simulink model "PMSM_simulink"  (R2023b)
settings: Solver=VariableStepAuto  StartTime=0.0  StopTime=15  RelTol=1e-3
undefined symbols (not defined in the file or in its folder): dyn, foc, fw, load, lut, org, pmsm, sigbuilder_block
libraries: slpidlib x3, eeTransforms x2
settings Model: Creator=MatlabStation  LastModifiedBy=arne.spiessens
settings OptimizationCC: ReuseModelBlockBuffer=off
settings DebuggingCC: AlgebraicLoopMsg=none  ParameterPrecisionLossMsg=none

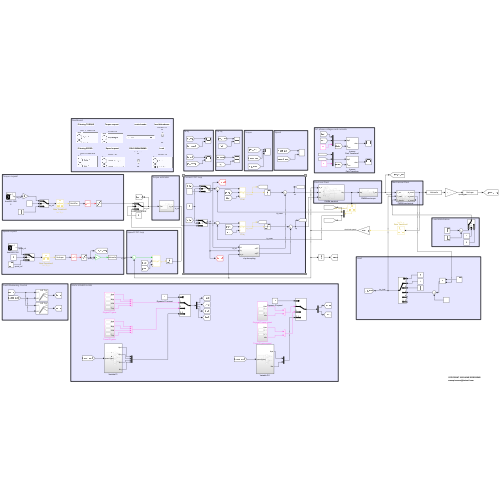
[thumbnail: Simulink's stored preview of the top-level diagram]
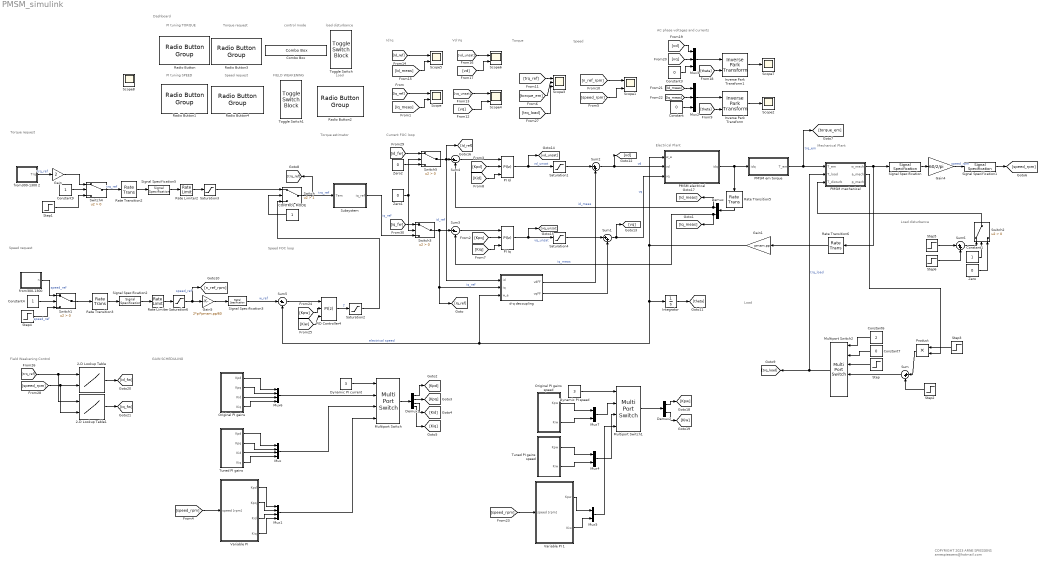
== system PMSM_simulink ==
  note: COPYRIGHT 2023 ARNE SPIESSENS
      | arnespiessens@hotmail.com
  note: Field Weakening Control
  note: Torque estimator
  note: Dashboard
  note: Load disturbance
  note: Speed FOC loop
  note: Speed request
  note: Torque request
  note: Current FOC loop
  note: Load
  note: GAIN SCHEDULING
  note: AC phase voltages and currents
  note: Speed
  note: Torque
  note: Vd Vq
  note: Id Iq
  note: Mechanical Plant
  note: Electrical Plant
  note: PI tuning TORQUE
  note: control mode
  note: PI tuning SPEED
  note: Torque request
  note: Speed request
  note: Load
  note: load disturbance
  note: FIELD WEAKENING
  2-D Lookup Table : Lookup_n-D  BreakpointsForDimension1=lut.trqLUT  BreakpointsForDimension2=lut.speedLUT  Table=lut.idLUT  InternalRulePriority=Speed  RndMeth=Simplest
      settings: InputPortMap=u0,u1
  2-D Lookup Table1 : Lookup_n-D  BreakpointsForDimension1=lut.trqLUT  BreakpointsForDimension2=lut.speedLUT  Table=lut.iqLUT  InternalRulePriority=Speed  RndMeth=Simplest
      settings: InputPortMap=u0,u1
  CONTROL MODE : Constant
  Combo Box : ComboBox  LabelPosition=Hide  SelectedLabel=Speed CL
      settings: Values={{'Torque CL', 'Speed CL'}, [2 1]}
  Constant : Constant  Value=0
  Constant1 : Constant
  Constant3 : Constant  Value=0
  Constant4 : Constant
  Constant6 : Constant  Value=2
  Constant7 : Constant  Value=0
  Constant9 : Constant
  Demux : Demux  Outputs=2
  Demux1 : Demux
  Demux2 : Demux  Outputs=2
  Dynamic PI current : Constant  Value=3
  Dynamic PI speed : Constant  Value=3
  Gain : Gain  Gain=2
  Gain1 : Gain  Gain=pmsm.pp
  Gain4 : Gain  Gain=60/2/pi
  Gain5 : Gain  Gain=2*pi*pmsm.pp/60
  Integrator : Integrator
  Inverse Park Transform : eeTransforms/Inverse Park Transform  AxisAlignment=Q-axis  PowerInvariant=off
      settings: LibrarySourceBlock=|
      | ee_sl_lib/Mathematical
      | Transforms/Inverse
      | Park Transform
  Inverse Park Transform1 : eeTransforms/Inverse Park Transform  AxisAlignment=Q-axis  PowerInvariant=off
      settings: LibrarySourceBlock=|
      | ee_sl_lib/Mathematical
      | Transforms/Inverse
      | Park Transform
  Multiport Switch : MultiPortSwitch  SaturateOnIntegerOverflow=off  InputSameDT=off
  Multiport Switch1 : MultiPortSwitch  SaturateOnIntegerOverflow=off  InputSameDT=off
  Multiport Switch2 : MultiPortSwitch  Inputs=5  SaturateOnIntegerOverflow=off  InputSameDT=off
  Mux : Mux
  Mux1 : Mux
  Mux2 : Mux  Inputs=3
  Mux3 : Mux  Inputs=3
  Mux4 : Mux  Inputs=2
  Mux5 : Mux  Inputs=2
  Mux6 : Mux
  Mux7 : Mux  Inputs=2
  Original PI gains : Subsystem
  Original PI gains speed : Subsystem
  PI Id : slpidlib/PID Controller  Controller=PI  Form=Parallel  TimeDomain=Discrete-time  UseExternalTs=off  SampleTime=foc.Ts_c  IntegratorMethod=Forward Euler  FilterMethod=Forward Euler  ControllerParametersSource=external  P=foc.Kpd  I=foc.Kid  UseKiTs=off  D=0  N=100  UseFilter=on  TunerSelectOption=Transfer Function Based (PID Tuner App)  InitialConditionSource=internal  InitialConditionForIntegrator=0  InitialConditionForFilter=0  DifferentiatorICPrevScaledInput=0  ExternalReset=none  TrackingMode=off  Kt=1  LimitOutput=on  SatLimitsSource=internal  UpperSaturationLimit=inf  LowerSaturationLimit=-inf  LinearizeAsGain=on  AntiWindupMode=clamping  Kb=foc.Kbd  LimitIntegrator=off  UpperIntegratorSaturationLimit=inf  LowerIntegratorSaturationLimit=-inf  POutMin=[]  POutMax=[]  IOutMin=[]  IOutMax=[]  DOutMin=[]  DOutMax=[]  NOutMin=[]  NOutMax=[]  SumOutMin=[]  SumOutMax=[]  SaturationOutMin=[]  SaturationOutMax=[]  PParamMin=[]  PParamMax=[]  IParamMin=[]  IParamMax=[]  DParamMin=[]  DParamMax=[]  NParamMin=[]  NParamMax=[]  KbParamMin=[]  KbParamMax=[]  KtParamMin=[]  KtParamMax=[]  KbOutMin=[]  KbOutMax=[]  KtOutMin=[]  KtOutMax=[]  IntegratorOutMin=[]  IntegratorOutMax=[]  FilterOutMin=[]  FilterOutMax=[]  SumI1OutMin=[]  SumI1OutMax=[]  SumI2OutMin=[]  SumI2OutMax=[]  SumI3OutMin=[]  SumI3OutMax=[]  SumI4OutMin=[]  SumI4OutMax=[]  SumDOutMin=[]  SumDOutMax=[]  DifferentiatorOutMin=[]  DifferentiatorOutMax=[]  FilterDiffOutCoefMin=[]  FilterDiffOutCoefMax=[]  ReciprocalOutMin=[]  ReciprocalOutMax=[]  SumDenOutMin=[]  SumDenOutMax=[]  SumNumOutMin=[]  SumNumOutMax=[]  DivideOutMin=[]  DivideOutMax=[]  UdiffTsProdOutMin=[]  UdiffTsProdOutMax=[]  NTsProdOutMin=[]  NTsProdOutMax=[]  UintegralTsProdOutMin=[]  UintegralTsProdOutMax=[]  UngainTsProdOutMin=[]  UngainTsProdOutMax=[]  ClampingZeroOutDataTypeStr=Inherit: Inherit via back propagation  ClampingZeroOutMin=[]  ClampingZeroOutMax=[]  FilterDenConstantOutDataTypeStr=Inherit: Inherit via back propagation  FilterDenConstantOutMin=[]  FilterDenConstantOutMax=[]  PCopyOutDataTypeStr=Inherit: Inherit via back propagation  PCopyOutMin=[]  PCopyOutMax=[]  NCopyOutDataTypeStr=Inherit: Inherit via back propagation  NCopyOutMin=[]  NCopyOutMax=[]  IntegratorContinuousStateAttributes=''  IntegratorStateMustResolveToSignalObject=off  IntegratorRTWStateStorageClass=Auto  FilterContinuousStateAttributes=''  FilterStateMustResolveToSignalObject=off  FilterRTWStateStorageClass=Auto  ParallelPVariant=ExternalParameters  IdealPVariant=Disabled  IVariant=ExternalParameters  DVariant=Disabled  IntegratorVariant=Discrete  SatVariant=Enabled  AWVariant=DiscClampingParallel  PCopyVariant=Disabled  TRVariant=Disabled  FdbkBlocksVariant=Forward  IdealPFdbkVariant=Disabled  SatFdbkVariant=Disabled  DerivativeFilterVariant=Disabled  NVariant=Disabled  NCopyVariant=Disabled_SignalSpec  FilterICVariant=Disabled  IntegratorICVariant=InternalICs  ExternalResetVariant=Disabled  TRSumVariant=Passthrough  SumFdbkVariant=Disabled  SumVariant=Sum_PI  TsampFilterVariant=InternalTs  TsampNgainVariant=Passthrough  TsampIntegralVariant=Disabled_SignalSpec  ExternalSaturationOutDataTypeStr=Inherit: Same as second input
  PI Iq : slpidlib/PID Controller  Controller=PI  Form=Parallel  TimeDomain=Discrete-time  UseExternalTs=off  SampleTime=foc.Ts_c  IntegratorMethod=Forward Euler  FilterMethod=Forward Euler  ControllerParametersSource=external  P=foc.Kpq  I=foc.Kiq  UseKiTs=off  D=0  N=100  UseFilter=on  TunerSelectOption=Transfer Function Based (PID Tuner App)  InitialConditionSource=internal  InitialConditionForIntegrator=0  InitialConditionForFilter=0  DifferentiatorICPrevScaledInput=0  ExternalReset=none  TrackingMode=off  Kt=1  LimitOutput=on  SatLimitsSource=internal  UpperSaturationLimit=inf  LowerSaturationLimit=-inf  LinearizeAsGain=on  AntiWindupMode=clamping  Kb=foc.Kbq  LimitIntegrator=off  UpperIntegratorSaturationLimit=inf  LowerIntegratorSaturationLimit=-inf  POutMin=[]  POutMax=[]  IOutMin=[]  IOutMax=[]  DOutMin=[]  DOutMax=[]  NOutMin=[]  NOutMax=[]  SumOutMin=[]  SumOutMax=[]  SaturationOutMin=[]  SaturationOutMax=[]  PParamMin=[]  PParamMax=[]  IParamMin=[]  IParamMax=[]  DParamMin=[]  DParamMax=[]  NParamMin=[]  NParamMax=[]  KbParamMin=[]  KbParamMax=[]  KtParamMin=[]  KtParamMax=[]  KbOutMin=[]  KbOutMax=[]  KtOutMin=[]  KtOutMax=[]  IntegratorOutMin=[]  IntegratorOutMax=[]  FilterOutMin=[]  FilterOutMax=[]  SumI1OutMin=[]  SumI1OutMax=[]  SumI2OutMin=[]  SumI2OutMax=[]  SumI3OutMin=[]  SumI3OutMax=[]  SumI4OutMin=[]  SumI4OutMax=[]  SumDOutMin=[]  SumDOutMax=[]  DifferentiatorOutMin=[]  DifferentiatorOutMax=[]  FilterDiffOutCoefMin=[]  FilterDiffOutCoefMax=[]  ReciprocalOutMin=[]  ReciprocalOutMax=[]  SumDenOutMin=[]  SumDenOutMax=[]  SumNumOutMin=[]  SumNumOutMax=[]  DivideOutMin=[]  DivideOutMax=[]  UdiffTsProdOutMin=[]  UdiffTsProdOutMax=[]  NTsProdOutMin=[]  NTsProdOutMax=[]  UintegralTsProdOutMin=[]  UintegralTsProdOutMax=[]  UngainTsProdOutMin=[]  UngainTsProdOutMax=[]  ClampingZeroOutDataTypeStr=Inherit: Inherit via back propagation  ClampingZeroOutMin=[]  ClampingZeroOutMax=[]  FilterDenConstantOutDataTypeStr=Inherit: Inherit via back propagation  FilterDenConstantOutMin=[]  FilterDenConstantOutMax=[]  PCopyOutDataTypeStr=Inherit: Inherit via back propagation  PCopyOutMin=[]  PCopyOutMax=[]  NCopyOutDataTypeStr=Inherit: Inherit via back propagation  NCopyOutMin=[]  NCopyOutMax=[]  IntegratorContinuousStateAttributes=''  IntegratorStateMustResolveToSignalObject=off  IntegratorRTWStateStorageClass=Auto  FilterContinuousStateAttributes=''  FilterStateMustResolveToSignalObject=off  FilterRTWStateStorageClass=Auto  ParallelPVariant=ExternalParameters  IdealPVariant=Disabled  IVariant=ExternalParameters  DVariant=Disabled  IntegratorVariant=Discrete  SatVariant=Enabled  AWVariant=DiscClampingParallel  PCopyVariant=Disabled  TRVariant=Disabled  FdbkBlocksVariant=Forward  IdealPFdbkVariant=Disabled  SatFdbkVariant=Disabled  DerivativeFilterVariant=Disabled  NVariant=Disabled  NCopyVariant=Disabled_SignalSpec  FilterICVariant=Disabled  IntegratorICVariant=InternalICs  ExternalResetVariant=Disabled  TRSumVariant=Passthrough  SumFdbkVariant=Disabled  SumVariant=Sum_PI  TsampFilterVariant=InternalTs  TsampNgainVariant=Passthrough  TsampIntegralVariant=Disabled_SignalSpec  ExternalSaturationOutDataTypeStr=Inherit: Same as second input
  PID Controller4 : slpidlib/PID Controller  Controller=PI  Form=Parallel  TimeDomain=Discrete-time  UseExternalTs=off  SampleTime=foc.Ts_s  IntegratorMethod=Forward Euler  FilterMethod=Forward Euler  ControllerParametersSource=external  P=foc.Kpw  I=foc.Kiw  UseKiTs=off  D=0  N=100  UseFilter=on  TunerSelectOption=Transfer Function Based (PID Tuner App)  InitialConditionSource=internal  InitialConditionForIntegrator=0  InitialConditionForFilter=0  DifferentiatorICPrevScaledInput=0  ExternalReset=none  TrackingMode=off  Kt=1  LimitOutput=on  SatLimitsSource=internal  UpperSaturationLimit=inf  LowerSaturationLimit=-inf  LinearizeAsGain=on  AntiWindupMode=clamping  Kb=foc.Kbw  LimitIntegrator=off  UpperIntegratorSaturationLimit=inf  LowerIntegratorSaturationLimit=-inf  POutMin=[]  POutMax=[]  IOutMin=[]  IOutMax=[]  DOutMin=[]  DOutMax=[]  NOutMin=[]  NOutMax=[]  SumOutMin=[]  SumOutMax=[]  SaturationOutMin=[]  SaturationOutMax=[]  PParamMin=[]  PParamMax=[]  IParamMin=[]  IParamMax=[]  DParamMin=[]  DParamMax=[]  NParamMin=[]  NParamMax=[]  KbParamMin=[]  KbParamMax=[]  KtParamMin=[]  KtParamMax=[]  KbOutMin=[]  KbOutMax=[]  KtOutMin=[]  KtOutMax=[]  IntegratorOutMin=[]  IntegratorOutMax=[]  FilterOutMin=[]  FilterOutMax=[]  SumI1OutMin=[]  SumI1OutMax=[]  SumI2OutMin=[]  SumI2OutMax=[]  SumI3OutMin=[]  SumI3OutMax=[]  SumI4OutMin=[]  SumI4OutMax=[]  SumDOutMin=[]  SumDOutMax=[]  DifferentiatorOutMin=[]  DifferentiatorOutMax=[]  FilterDiffOutCoefMin=[]  FilterDiffOutCoefMax=[]  ReciprocalOutMin=[]  ReciprocalOutMax=[]  SumDenOutMin=[]  SumDenOutMax=[]  SumNumOutMin=[]  SumNumOutMax=[]  DivideOutMin=[]  DivideOutMax=[]  UdiffTsProdOutMin=[]  UdiffTsProdOutMax=[]  NTsProdOutMin=[]  NTsProdOutMax=[]  UintegralTsProdOutMin=[]  UintegralTsProdOutMax=[]  UngainTsProdOutMin=[]  UngainTsProdOutMax=[]  ClampingZeroOutDataTypeStr=Inherit: Inherit via back propagation  ClampingZeroOutMin=[]  ClampingZeroOutMax=[]  FilterDenConstantOutDataTypeStr=Inherit: Inherit via back propagation  FilterDenConstantOutMin=[]  FilterDenConstantOutMax=[]  PCopyOutDataTypeStr=Inherit: Inherit via back propagation  PCopyOutMin=[]  PCopyOutMax=[]  NCopyOutDataTypeStr=Inherit: Inherit via back propagation  NCopyOutMin=[]  NCopyOutMax=[]  IntegratorContinuousStateAttributes=''  IntegratorStateMustResolveToSignalObject=off  IntegratorRTWStateStorageClass=Auto  FilterContinuousStateAttributes=''  FilterStateMustResolveToSignalObject=off  FilterRTWStateStorageClass=Auto  ParallelPVariant=ExternalParameters  IdealPVariant=Disabled  IVariant=ExternalParameters  DVariant=Disabled  IntegratorVariant=Discrete  SatVariant=Enabled  AWVariant=DiscClampingParallel  PCopyVariant=Disabled  TRVariant=Disabled  FdbkBlocksVariant=Forward  IdealPFdbkVariant=Disabled  SatFdbkVariant=Disabled  DerivativeFilterVariant=Disabled  NVariant=Disabled  NCopyVariant=Disabled_SignalSpec  FilterICVariant=Disabled  IntegratorICVariant=InternalICs  ExternalResetVariant=Disabled  TRSumVariant=Passthrough  SumFdbkVariant=Disabled  SumVariant=Sum_PI  TsampFilterVariant=InternalTs  TsampNgainVariant=Passthrough  TsampIntegralVariant=Disabled_SignalSpec  ExternalSaturationOutDataTypeStr=Inherit: Same as second input
  PMSM electrical : Subsystem
  PMSM em torque : Subsystem
  PMSM mechanical : Subsystem
  Product : Product
  Radio Button : RadioButtonGroup  SelectedLabel=Dynamic scheduling  ButtonGroupName=Group
      settings: Values={{'Original PI', 'Tuned PI', 'Dynamic scheduling'}, [1 2 3]}
  Radio Button1 : RadioButtonGroup  SelectedLabel=Dynamic scheduling  ButtonGroupName=Group
      settings: Values={{'Original PI', 'Tuned PI', 'Dynamic scheduling'}, [1 2 3]}
  Radio Button2 : RadioButtonGroup  SelectedLabel=Friction load  ButtonGroupName=Group
      settings: Values={{'No load', 'Friction load', 'Friction + inertia load'}, [1 2 3]}
  Radio Button3 : RadioButtonGroup  SelectedLabel=TRQ dynamic request  ButtonGroupName=Group
      settings: Values={{'TRQ step request', 'TRQ dynamic request'}, [0 1]}
  Radio Button4 : RadioButtonGroup  SelectedLabel=SPEED dynamic request  ButtonGroupName=Group
      settings: Values={{'SPEED step request', 'SPEED dynamic request'}, [0 1]}
  Rate Limiter : RateLimiter  RisingSlewLimit=foc.slew_speed  FallingSlewLimit=-foc.slew_speed  SampleTimeMode=inherited
  Rate Limiter2 : RateLimiter  RisingSlewLimit=foc.slew_torque  FallingSlewLimit=-foc.slew_torque  SampleTimeMode=inherited
  Rate Transition2 : RateTransition  OutPortSampleTime=foc.Ts_c
      settings: AttributesFormatString=%<OutPortSampleTime>
  Rate Transition3 : RateTransition  OutPortSampleTime=foc.Ts_s
      settings: AttributesFormatString=%<OutPortSampleTime>
  Rate Transition5 : RateTransition  OutPortSampleTime=foc.Ts_c
      settings: AttributesFormatString=%<OutPortSampleTime>
  Rate Transition6 : RateTransition  OutPortSampleTime=foc.Ts_s
      settings: AttributesFormatString=%<OutPortSampleTime>
  Saturation1 : Saturate  UpperLimit=fw.vs_max  LowerLimit=-fw.vs_max
  Saturation2 : Saturate  UpperLimit=fw.trq_max  LowerLimit=-fw.trq_max
  Saturation3 : Saturate  UpperLimit=fw.trq_max  LowerLimit=-fw.trq_max
  Saturation4 : Saturate  UpperLimit=fw.vs_max  LowerLimit=-fw.vs_max
  Saturation6 : Saturate  UpperLimit=pmsm.n_rat  LowerLimit=-pmsm.n_rat
  Scope{,1,4..6} (5 alike) : Scope  NumInputPorts=2
  Scope2 : Scope
  Scope3 : Scope  NumInputPorts=3
  Scope7 : Scope
  Signal Specification : SignalSpecification  Unit=rad/s
  Signal Specification1 : SignalSpecification  Unit=rpm
  Signal Specification2 : SignalSpecification  Unit=rpm
  Signal Specification3 : SignalSpecification  Unit=rad/s
  Signal Specification5 : SignalSpecification  Unit=N*m
  Step : Step  After=load.trq_f  SampleTime=0
  Step1 : Step  After=fw.trq_max  SampleTime=0
  Step2 : Step  After=load.trq_f  SampleTime=0
  Step3 : Step  After=load.J  SampleTime=0
  Step4 : Step  After=440  SampleTime=0
  Step5 : Step  Time=2  After=3  SampleTime=0
  Step6 : Step  Time=2.05  After=-3  SampleTime=0
  Subsystem : Subsystem
  Sum{,1..2,6} (4 alike) : Sum  Inputs=|++
  Sum3 : Sum  Inputs=|+-
  Sum4 : Sum  Inputs=|+-
  Sum5 : Sum  Inputs=|+-
  Switch : Switch  Criteria=u2 > Threshold  Threshold=1  SaturateOnIntegerOverflow=off  InputSameDT=off
  Switch{1..5} (5 alike) : Switch  Criteria=u2 > Threshold  SaturateOnIntegerOverflow=off  InputSameDT=off
  Toggle Switch : ToggleSwitchBlock
      settings: Values={{'Off', 'On'}, [0 1]}
  Toggle Switch1 : ToggleSwitchBlock
      settings: Values={{'Off', 'On'}, [0 1]}
  Tuned PI gains : Subsystem
  Tuned PI gains speed : Subsystem
  "Variable PI " : Subsystem
  Variable PI 1 : Subsystem
  Zero : Constant  Value=0  OutDataTypeStr=Inherit: Inherit via back propagation
  Zero1 : Constant  Value=0  OutDataTypeStr=Inherit: Inherit via back propagation
  Zero2 : Constant  Value=0  OutDataTypeStr=Inherit: Inherit via back propagation
  d-q decoupling : Subsystem
  "from300-1300 " : Subsystem  Tag=STV Subsys  LoadFcn=sigbuilder_block('load');  StartFcn=sigbuilder_block('start');  StopFcn=sigbuilder_block('stop');  ClipboardFcn=sigbuilder_block('clipboard');  mask(Sigbuilder block){tuvar=[0:10]}
      mask help: Sigbuilder GUI
      mask init:
      | if ~strcmp(get_param(bdroot(gcbh),'SimulationStatus'),'stopped') tuvar = sigbuilder_block('maskInit'); end
      settings: CopyFcn=sigbuilder_block('copy');  DeleteFcn=sigbuilder_block('delete');  ModelCloseFcn=sigbuilder_block('modelClose');  PreSaveFcn=sigbuilder_block('preSave');  PauseFcn=sigbuilder_block('pause')  ContinueFcn=sigbuilder_block('continue')  NameChangeFcn=sigbuilder_block('namechange');  OpenFcn=sigbuilder_block('open',[6 6 948 470.25 ]);  CloseFcn=sigbuilder_block('close');
      mask Display: plot(0, 0, 100, 100,[2, 2, 32, 32, 2], [68, 8, 8, 68, 68],[32, 2], [38, 38], [32, 19, 2],[53, 60, 44], [32, 17, 17, 2],[16, 16, 31, 31]);txt = getActiveGroup(gcbh);text(2, 100, txt,'verticalAlignment', 'top');
  from300-1300 2 : Subsystem  Tag=STV Subsys  LoadFcn=sigbuilder_block('load');  StartFcn=sigbuilder_block('start');  StopFcn=sigbuilder_block('stop');  ClipboardFcn=sigbuilder_block('clipboard');  mask(Sigbuilder block){tuvar=[0:10]}
      mask help: Sigbuilder GUI
      mask init:
      | if ~strcmp(get_param(bdroot(gcbh),'SimulationStatus'),'stopped') tuvar = sigbuilder_block('maskInit'); end
      settings: CopyFcn=sigbuilder_block('copy');  DeleteFcn=sigbuilder_block('delete');  ModelCloseFcn=sigbuilder_block('modelClose');  PreSaveFcn=sigbuilder_block('preSave');  PauseFcn=sigbuilder_block('pause')  ContinueFcn=sigbuilder_block('continue')  NameChangeFcn=sigbuilder_block('namechange');  OpenFcn=sigbuilder_block('open',[6 46.2 948 430.05 ]);  CloseFcn=sigbuilder_block('close');
      mask Display: plot(0, 0, 100, 100,[2, 2, 32, 32, 2], [68, 8, 8, 68, 68],[32, 2], [38, 38], [32, 19, 2],[53, 60, 44], [32, 17, 17, 2],[16, 16, 31, 31]);txt = getActiveGroup(gcbh);text(2, 100, txt,'verticalAlignment', 'top');
  Scope8 : Scope
  wires:
  Switch4/1 -> Rate Transition2/1  "trq_ref"
  Switch3/1 -> Sum3/1, d-q decoupling/2(iq), [Iq_ref]  "iq_ref"
  Demux/1 -> [Id_meas], Sum4/2  "id_meas"
  Constant/1 -> Mux2/3
  Integrator/1 -> [theta]
  Switch5/1 -> [Id_ref], d-q decoupling/1(id), Sum4/1  "id_ref"
  Mux2/1 -> Inverse Park Transform/1
  Gain1/1 -> PMSM electrical/1(w_e), d-q decoupling/3(w_e), Sum5/2, Integrator/1  "electrical speed"
  [theta] -> Inverse Park Transform/2
  "Variable PI "/4(Kiq) -> Mux1/4
  Signal Specification/1 -> Gain4/1
  [Iq_meas] -> Scope/2
  [Kpd] -> PI Id/2
  [Iq_ref] -> Scope/1
  "Variable PI "/1(Kpd) -> Mux1/1
  Sum1/1 -> PMSM electrical/3(vq), [vq]  "vq"
  Saturation1/1 -> Sum2/1
  PMSM em torque/1(T_em) -> [torque_em], PMSM mechanical/1(T_em)  "trq_em"
  PMSM electrical/1(idq) -> Rate Transition5/1, PMSM em torque/1(idq)
  Signal Specification1/1 -> [speed_rpm]
  [n_ref_rpm] -> Scope1/1
  Sum4/1 -> PI Id/1
  Saturation2/1 -> Switch/3
  "Variable PI "/3(Kid) -> Mux1/3
  [torque_em] -> Scope3/2
  "Variable PI "/2(Kpq) -> Mux1/2
  [Kiq] -> PI Iq/3
  [vq_unsat] -> Scope4/1
  Rate Limiter2/1 -> Saturation3/1
  d-q decoupling/1(vdFF) -> Sum2/2
  Multiport Switch2/1 -> PMSM mechanical/2(T_load), [trq_load]  "trq_load"
  Inverse Park Transform/1 -> Scope2/1
  Signal Specification5/1 -> Rate Limiter2/1
  Gain5/1 -> Signal Specification3/1
  Rate Transition3/1 -> Signal Specification2/1
  Rate Transition2/1 -> Signal Specification5/1
  Demux/2 -> [Iq_meas], Sum3/2  "iq_meas"
  PI Id/1 -> [vd_unsat], Saturation1/1  "vd_unsat"
  Rate Transition6/1 -> Gain1/1
  Sum5/1 -> PID Controller4/1
  PI Iq/1 -> Saturation4/1, [vq_unsat]  "vq_unsat"
  PID Controller4/1 -> Saturation2/1  "T"
  Rate Transition5/1 -> Demux/1
  Signal Specification3/1 -> Sum5/1  "w_ref"
  [speed_rpm] -> "Variable PI "/1(speed [rpm])
  [Kpq] -> PI Iq/2
  Signal Specification2/1 -> Rate Limiter/1
  [speed_rpm] -> Scope1/2
  [trq_ref] -> Scope3/1
  Mux1/1 -> Multiport Switch/4
  [Kid] -> PI Id/3
  CONTROL MODE/1 -> Switch/2
  Gain4/1 -> Signal Specification1/1  "speed_rpm"
  [vq] -> Scope4/2
  d-q decoupling/2(vqFF) -> Sum1/2
  Sum2/1 -> PMSM electrical/2(vd), [vd]  "vd"
  Rate Limiter/1 -> Saturation6/1
  Sum3/1 -> PI Iq/1
  [Id_ref] -> Scope5/1
  [Id_meas] -> Scope5/2
  [vd] -> Scope6/2
  [vd_unsat] -> Scope6/1
  [theta] -> Inverse Park Transform1/2
  Mux3/1 -> Inverse Park Transform1/1
  [vd] -> Mux3/1
  Inverse Park Transform1/1 -> Scope7/1
  Constant3/1 -> Mux3/3
  [vq] -> Mux3/2
  [Id_meas] -> Mux2/1
  [Iq_meas] -> Mux2/2
  Saturation4/1 -> Sum1/1
  Saturation6/1 -> [n_ref_rpm], Gain5/1  "speed_ref"
  Tuned PI gains speed/1(Kpw) -> Mux4/1
  Multiport Switch1/1 -> Demux2/1
  Demux2/2 -> [Kiw]
  Demux2/1 -> [Kpw]
  Variable PI 1/1(Kpw) -> Mux5/1
  Mux5/1 -> Multiport Switch1/4
  [speed_rpm] -> Variable PI 1/1(speed [rpm])
  Tuned PI gains speed/2(Kiw) -> Mux4/2
  Dynamic PI speed/1 -> Multiport Switch1/1
  Variable PI 1/2(Kiw) -> Mux5/2
  [Kpw] -> PID Controller4/2
  [Kiw] -> PID Controller4/3
  Demux1/4 -> [Kiq]
  Demux1/1 -> [Kpd]
  Demux1/3 -> [Kid]
  Demux1/2 -> [Kpq]
  Multiport Switch/1 -> Demux1/1
  Dynamic PI current/1 -> Multiport Switch/1
  Original PI gains/1(Kpd) -> Mux6/1
  Original PI gains/2(Kpq) -> Mux6/2
  Original PI gains/3(Kid) -> Mux6/3
  Mux6/1 -> Multiport Switch/2
  Original PI gains/4(Kiq) -> Mux6/4
  Mux/1 -> Multiport Switch/3
  Tuned PI gains/4(Kiq) -> Mux/4
  Tuned PI gains/1(Kpd) -> Mux/1
  Tuned PI gains/2(Kpq) -> Mux/2
  Tuned PI gains/3(Kid) -> Mux/3
  Mux7/1 -> Multiport Switch1/2
  Original PI gains speed/1(Kpw) -> Mux7/1
  Original PI gains speed/2(Kiw) -> Mux7/2
  Mux4/1 -> Multiport Switch1/3
  Constant6/1 -> Multiport Switch2/1
  Constant7/1 -> Multiport Switch2/2
  Step/1 -> Multiport Switch2/3
  [trq_load] -> Scope3/3
  Step1/1 -> Switch4/3
  from300-1300 2/1(Trq) -> Gain/1  "trq_ref"
  Constant9/1 -> Switch4/2
  Step2/1 -> Sum/2
  Sum/1 -> Multiport Switch2/4
  Product/1 -> Sum/1
  Step3/1 -> Product/1
  PMSM mechanical/2(a_mech) -> Product/2
  PMSM mechanical/1(w_mech) -> Rate Transition6/1, Signal Specification/1
  Switch1/1 -> Rate Transition3/1
  Constant4/1 -> Switch1/2
  "from300-1300 "/1(n) -> Switch1/1  "speed_ref"
  Step4/1 -> Switch1/3  "speed_ref"
  Switch2/1 -> PMSM mechanical/3(T_disturb)
  Gain/1 -> Switch4/1
  Step5/1 -> Sum6/1
  Step6/1 -> Sum6/2
  Sum6/1 -> Switch2/1
  Zero/1 -> Switch2/3
  Constant1/1 -> Switch2/2
  Saturation3/1 -> Switch/1
  2-D Lookup Table/1 -> [id_fw]
  2-D Lookup Table1/1 -> [iq_fw]
  [trq_ref] -> 2-D Lookup Table1/1, 2-D Lookup Table/1
  [speed_rpm] -> 2-D Lookup Table1/2, 2-D Lookup Table/2
  Zero2/1 -> Switch5/3
  [id_fw] -> Switch5/1
  Switch/1 -> Subsystem/1(Tem), [trq_ref]  "trq_ref"
  Subsystem/1(iq_ref) -> Switch3/3  "iq_ref"
  Zero1/1 -> Switch3/2, Switch5/2
  [iq_fw] -> Switch3/1

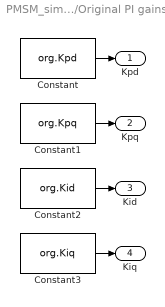
== system PMSM_simulink/Original PI gains ==
  Constant : Constant  Value=org.Kpd
  Constant1 : Constant  Value=org.Kpq
  Constant2 : Constant  Value=org.Kid
  Constant3 : Constant  Value=org.Kiq
  Kpd : Outport
  Kpq : Outport  Port=2
  Kid : Outport  Port=3
  Kiq : Outport  Port=4
  wires:
  Constant3/1 -> Kiq/1
  Constant1/1 -> Kpq/1
  Constant/1 -> Kpd/1
  Constant2/1 -> Kid/1

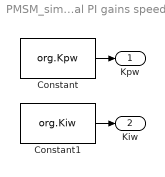
== system PMSM_simulink/Original PI gains speed ==
  Constant : Constant  Value=org.Kpw
  Constant1 : Constant  Value=org.Kiw
  Kpw : Outport
  Kiw : Outport  Port=2
  wires:
  Constant1/1 -> Kiw/1
  Constant/1 -> Kpw/1

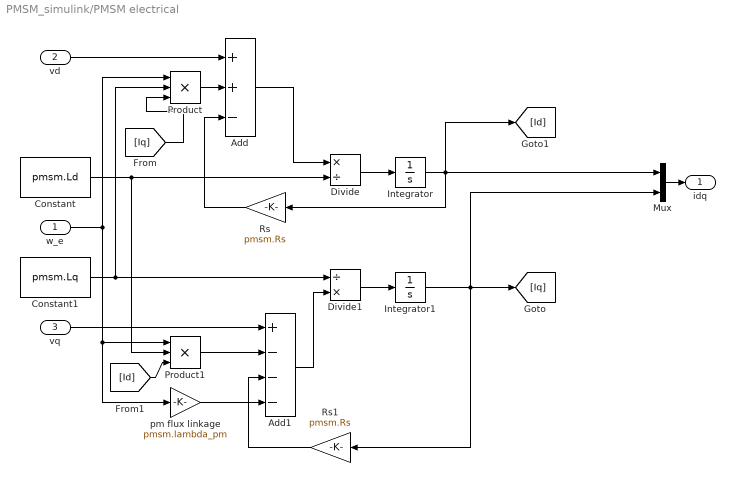
== system PMSM_simulink/PMSM electrical ==
  w_e : Inport
  vd : Inport  Port=2
  vq : Inport  Port=3
  Add : Sum  Inputs=++-
  Add1 : Sum  Inputs=+---
  Constant : Constant  Value=pmsm.Ld
  Constant1 : Constant  Value=pmsm.Lq
  Divide : Product  Inputs=*/
  Divide1 : Product  Inputs=/*
  Integrator : Integrator
  Integrator1 : Integrator
  Mux : Mux  Inputs=2
  Product : Product  Inputs=3
  Product1 : Product  Inputs=3
  Rs : Gain  Gain=pmsm.Rs
  Rs1 : Gain  Gain=pmsm.Rs
  pm flux linkage : Gain  Gain=pmsm.lambda_pm
  idq : Outport
  wires:
  Constant/1 -> Product1/2, Divide/2
  w_e/1 -> pm flux linkage/1, Product1/1, Product/1
  Constant1/1 -> Product/2, Divide1/1
  Product/1 -> Add/2
  Integrator/1 -> Rs/1, Mux/1, [Id]
  Rs/1 -> Add/3
  Add/1 -> Divide/1
  Divide/1 -> Integrator/1
  Integrator1/1 -> Rs1/1, [Iq], Mux/2
  Rs1/1 -> Add1/3
  Product1/1 -> Add1/2
  Divide1/1 -> Integrator1/1
  Add1/1 -> Divide1/2
  pm flux linkage/1 -> Add1/4
  Mux/1 -> idq/1
  [Iq] -> Product/3
  [Id] -> Product1/3
  vq/1 -> Add1/1
  vd/1 -> Add/1

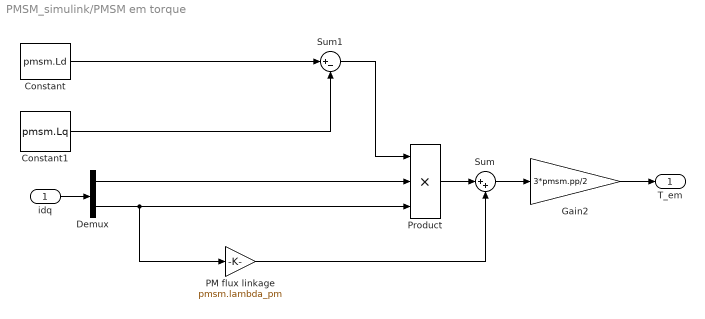
== system PMSM_simulink/PMSM em torque ==
  idq : Inport
  Constant : Constant  Value=pmsm.Ld
  Constant1 : Constant  Value=pmsm.Lq
  Demux : Demux  Outputs=2
  Gain2 : Gain  Gain=3*pmsm.pp/2
  PM flux linkage : Gain  Gain=pmsm.lambda_pm
  Product : Product  Inputs=3
  Sum : Sum  Inputs=|++
  Sum1 : Sum  Inputs=|+-
  T_em : Outport  VectorParamsAs1DForOutWhenUnconnected=off
  wires:
  Constant/1 -> Sum1/1
  Constant1/1 -> Sum1/2
  Demux/2 -> PM flux linkage/1, Product/3
  Product/1 -> Sum/1
  Sum/1 -> Gain2/1
  PM flux linkage/1 -> Sum/2
  Gain2/1 -> T_em/1
  idq/1 -> Demux/1
  Sum1/1 -> Product/1
  Demux/1 -> Product/2

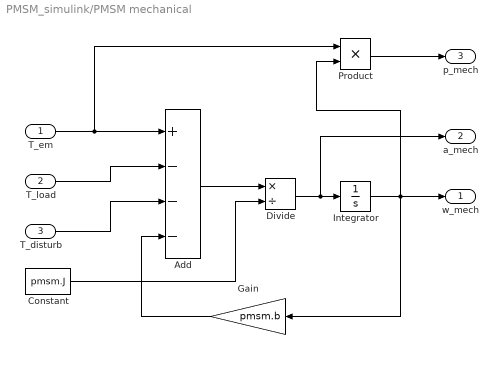
== system PMSM_simulink/PMSM mechanical ==
  T_em : Inport
  T_load : Inport  Port=2
  T_disturb : Inport  Port=3
  Add : Sum  Inputs=+---
  Constant : Constant  Value=pmsm.J
  Divide : Product  Inputs=*/
  Gain : Gain  Gain=pmsm.b
  Integrator : Integrator
  Product : Product
  w_mech : Outport
  a_mech : Outport  Port=2
  p_mech : Outport  Port=3
  wires:
  T_em/1 -> Product/1, Add/1
  T_load/1 -> Add/2
  Add/1 -> Divide/1
  Constant/1 -> Divide/2
  Divide/1 -> a_mech/1, Integrator/1
  Gain/1 -> Add/4
  Integrator/1 -> Product/2, w_mech/1, Gain/1
  T_disturb/1 -> Add/3
  Product/1 -> p_mech/1

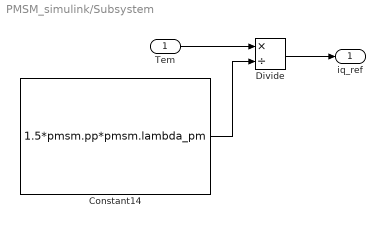
== system PMSM_simulink/Subsystem ==
  Tem : Inport
  Constant14 : Constant  Value=1.5*pmsm.pp*pmsm.lambda_pm  OutDataTypeStr=single
  Divide : Product  Inputs=*/
  iq_ref : Outport
  wires:
  Tem/1 -> Divide/1
  Constant14/1 -> Divide/2
  Divide/1 -> iq_ref/1

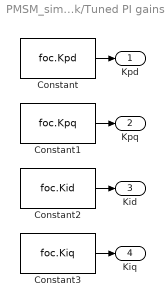
== system PMSM_simulink/Tuned PI gains ==
  Constant : Constant  Value=foc.Kpd
  Constant1 : Constant  Value=foc.Kpq
  Constant2 : Constant  Value=foc.Kid
  Constant3 : Constant  Value=foc.Kiq
  Kpd : Outport
  Kpq : Outport  Port=2
  Kid : Outport  Port=3
  Kiq : Outport  Port=4
  wires:
  Constant3/1 -> Kiq/1
  Constant1/1 -> Kpq/1
  Constant/1 -> Kpd/1
  Constant2/1 -> Kid/1

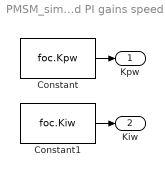
== system PMSM_simulink/Tuned PI gains speed ==
  Constant : Constant  Value=foc.Kpw
  Constant1 : Constant  Value=foc.Kiw
  Kpw : Outport
  Kiw : Outport  Port=2
  wires:
  Constant1/1 -> Kiw/1
  Constant/1 -> Kpw/1

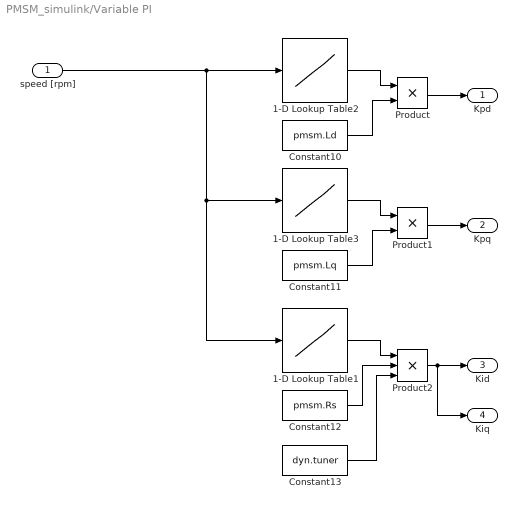
== system PMSM_simulink/Variable PI  ==
  speed [rpm] : Inport
  1-D Lookup Table1 : Lookup_n-D  NumberOfTableDimensions=1  BreakpointsForDimension1=dyn.speedVec_rpm  Table=dyn.bwVec_i_radps  InternalRulePriority=Speed  RndMeth=Simplest
  1-D Lookup Table2 : Lookup_n-D  NumberOfTableDimensions=1  BreakpointsForDimension1=dyn.speedVec_rpm  Table=dyn.bwVec_i_radps  InternalRulePriority=Speed  RndMeth=Simplest
  1-D Lookup Table3 : Lookup_n-D  NumberOfTableDimensions=1  BreakpointsForDimension1=dyn.speedVec_rpm  Table=dyn.bwVec_i_radps  InternalRulePriority=Speed  RndMeth=Simplest
  Constant10 : Constant  Value=pmsm.Ld
  Constant11 : Constant  Value=pmsm.Lq
  Constant12 : Constant  Value=pmsm.Rs
  Constant13 : Constant  Value=dyn.tuner
  Product : Product
  Product1 : Product
  Product2 : Product  Inputs=3
  Kpd : Outport
  Kpq : Outport  Port=2
  Kid : Outport  Port=3
  Kiq : Outport  Port=4
  wires:
  1-D Lookup Table2/1 -> Product/1
  Constant13/1 -> Product2/3
  Constant12/1 -> Product2/2
  1-D Lookup Table1/1 -> Product2/1
  1-D Lookup Table3/1 -> Product1/1
  Constant11/1 -> Product1/2
  Constant10/1 -> Product/2
  speed [rpm]/1 -> 1-D Lookup Table2/1, 1-D Lookup Table1/1, 1-D Lookup Table3/1
  Product/1 -> Kpd/1
  Product1/1 -> Kpq/1
  Product2/1 -> Kiq/1, Kid/1

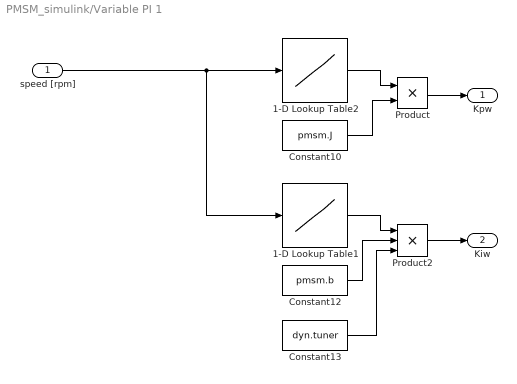
== system PMSM_simulink/Variable PI 1 ==
  speed [rpm] : Inport
  1-D Lookup Table1 : Lookup_n-D  NumberOfTableDimensions=1  BreakpointsForDimension1=dyn.speedVec_rpm  Table=dyn.bwVec_w_radps  InternalRulePriority=Speed  RndMeth=Simplest
  1-D Lookup Table2 : Lookup_n-D  NumberOfTableDimensions=1  BreakpointsForDimension1=dyn.speedVec_rpm  Table=dyn.bwVec_w_radps  InternalRulePriority=Speed  RndMeth=Simplest
  Constant10 : Constant  Value=pmsm.J
  Constant12 : Constant  Value=pmsm.b
  Constant13 : Constant  Value=dyn.tuner
  Product : Product
  Product2 : Product  Inputs=3
  Kpw : Outport
  Kiw : Outport  Port=2
  wires:
  1-D Lookup Table2/1 -> Product/1
  Constant13/1 -> Product2/3
  Constant12/1 -> Product2/2
  1-D Lookup Table1/1 -> Product2/1
  Constant10/1 -> Product/2
  speed [rpm]/1 -> 1-D Lookup Table2/1, 1-D Lookup Table1/1
  Product/1 -> Kpw/1
  Product2/1 -> Kiw/1

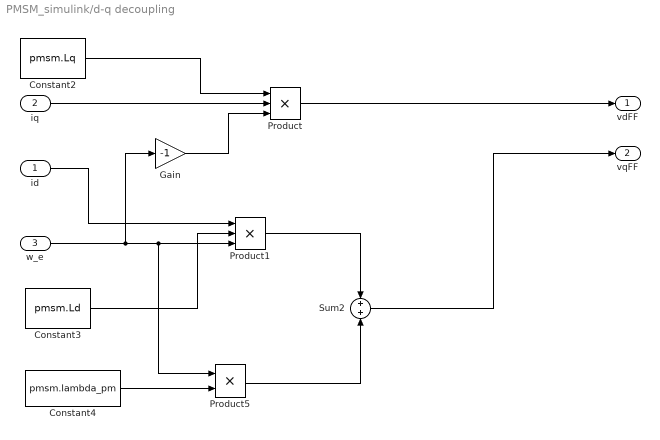
== system PMSM_simulink/d-q decoupling ==
  id : Inport
  iq : Inport  Port=2
  w_e : Inport  Port=3
  Constant2 : Constant  Value=pmsm.Lq
  Constant3 : Constant  Value=pmsm.Ld
  Constant4 : Constant  Value=pmsm.lambda_pm
  Gain : Gain  Gain=-1
  Product : Product  Inputs=3
  Product1 : Product  Inputs=3
  Product5 : Product
  Sum2 : Sum
  vdFF : Outport  VectorParamsAs1DForOutWhenUnconnected=off
  vqFF : Outport  Port=2  VectorParamsAs1DForOutWhenUnconnected=off
  wires:
  Sum2/1 -> vqFF/1
  Product/1 -> vdFF/1
  iq/1 -> Product/2
  Constant2/1 -> Product/1
  w_e/1 -> Product5/1, Product1/3, Gain/1
  id/1 -> Product1/1
  Constant3/1 -> Product1/2
  Constant4/1 -> Product5/2
  Product1/1 -> Sum2/1
  Product5/1 -> Sum2/2
  Gain/1 -> Product/3

== system PMSM_simulink/from300-1300  ==
  Demux : Demux  Tag=STV Demux  Outputs=1
      settings: DisplayOption=none
  FromWs : FromWorkspace  Tag=STV FromWs  VariableName=tuvar
      SigBuilderData=|
      | common.afterFinalStr = 'Extrapolate'
      | common.sampleTime = 0
      | dataSet.timeRange = [0 15]
      | dataSet.name = 'Group 1'
      | sbobj.Groups.Name = 'Group 1'
      | sbobj.Groups.Signals.Name = 'n'
      | sbobj.Groups.Signals.XData = [0 1 1 3 3 4 4 5 5 7 7 9 9 12 12 15]
      | sbobj.Groups.Signals.YData = [0 0 1000 1000 300 300 1500 1500 2500 2500 1000 1000 3000 3000 0 0]
      | sbobj.Groups.TimeRange = [0 15]
  n : Outport  Tag=STV Outport  VectorParamsAs1DForOutWhenUnconnected=off
  wires:
  Demux/1 -> n/1
  FromWs/1 -> Demux/1

== system PMSM_simulink/from300-1300 2 ==
  Demux : Demux  Tag=STV Demux  Outputs=1
      settings: DisplayOption=none
  FromWs : FromWorkspace  Tag=STV FromWs  VariableName=tuvar
      SigBuilderData=|
      | common.afterFinalStr = 'Extrapolate'
      | common.sampleTime = 0
      | dataSet.timeRange = [0 15]
      | dataSet.name = 'Group 1'
      | sbobj.Groups.Name = 'Group 1'
      | sbobj.Groups.Signals.Name = 'Trq'
      | sbobj.Groups.Signals.XData = [0 1 1 3 3 4 4 6 6 7.74 7.74 9 9 11 11 13 13 15]
      | sbobj.Groups.Signals.YData = [0 0 0.5 0.5 0 0 1 1 0 0 2 2 0 0 1.5 1.5 0 0]
      | sbobj.Groups.TimeRange = [0 15]
  Trq : Outport  Tag=STV Outport  VectorParamsAs1DForOutWhenUnconnected=off
  wires:
  Demux/1 -> Trq/1
  FromWs/1 -> Demux/1
